simulink model "CruiseControl_System"  (R2022b)
settings: Solver=VariableStepAuto  StartTime=0.0  StopTime=100  MaxStep=0.1  RelTol=1e-3
settings Model: Creator=MAAM  LastModifiedBy=MAAM

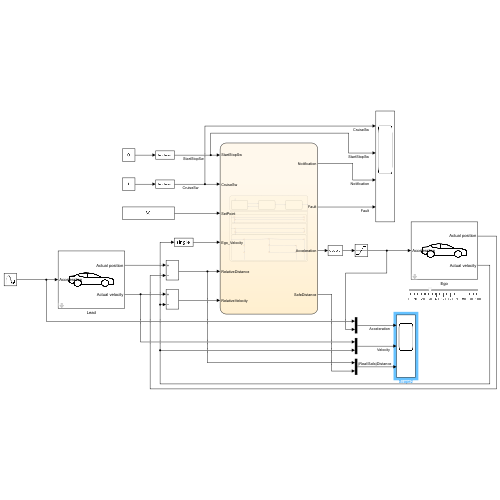
[thumbnail: Simulink's stored preview of the top-level diagram]
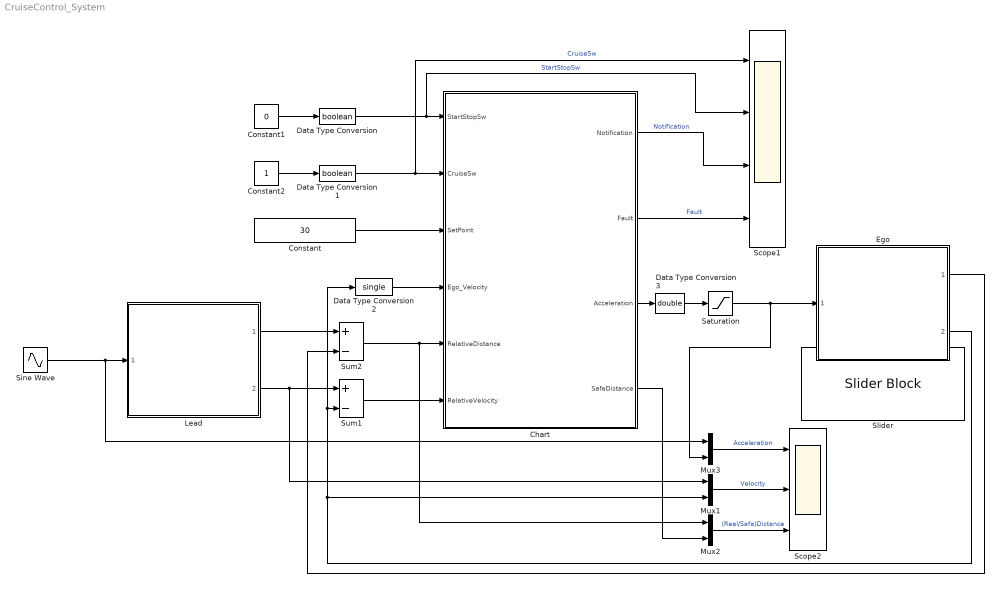
== system CruiseControl_System ==
  Chart : Stateflow chart  TreatAsAtomicUnit=on
      settings: PortSchema="{\"entries\":[{\"content\":{\"sides\":[{\"content\":{\"connectorIds\":[\"In2\",\"In1\",\"In3\",\"In4\",\"In5\",\"In6\"]},\"type\":\"ConnectorPlacement.EquallySpacedRectSide\",\"uuid\":\"a558f2c2-5ffb-4ba0-8891-a688bb62a9b9\"},{\"content\":{\"connectorIds\":[\"Out2\",\"Out1\",\"Out3\",\"Out4\"],\"side\":\"RIGHT\"},\"type\":\"ConnectorPlacement.EquallySpacedRectSide\",\"uuid\":\"56d0d55d-a484-4316-a2b8-f7c2ba28bad9\"},{\"content\":{\"connectorIds\":[],\"side\":\"TOP\"},\"type\":\"ConnectorPlacement.EquallySpacedRectSide\",\"uuid\":\"4bb91777-42b4-417b-88ce-c76e908bf247\"}]},\"type\":\"ConnectorPlacement.EquallySpacedConnector\",\"uuid\":\"a190dafd-ffc5-4ff1-968b-a32c0c19da50\"}],\"packageUris\":[\"http://schema.mathworks.com/mf0/Connector/R2020b\"],\"version\":\"1.0\"}"
  Constant : Constant  Value=30  OutDataTypeStr=single
  Constant1 : Constant  Value=0
  Constant2 : Constant
  Data Type Conversion : DataTypeConversion  OutDataTypeStr=boolean  SaturateOnIntegerOverflow=off  RndMeth=Floor
  Data Type Conversion1 : DataTypeConversion  OutDataTypeStr=boolean  SaturateOnIntegerOverflow=off  RndMeth=Floor
  Data Type Conversion2 : DataTypeConversion  OutDataTypeStr=single  SaturateOnIntegerOverflow=off  RndMeth=Floor
  Data Type Conversion3 : DataTypeConversion  OutDataTypeStr=double  SaturateOnIntegerOverflow=off  RndMeth=Floor
  Ego : Subsystem  ReferencedSubsystem=Car  InitPos=10  InitVol=20
  Lead : Subsystem  ReferencedSubsystem=Car  InitPos=50  InitVol=25
  Mux1 : Mux  Inputs=2
  Mux2 : Mux  Inputs=2
  Mux3 : Mux  Inputs=2
  Saturation : Saturate  UpperLimit=2  LowerLimit=-3
  Scope1 : Scope  NumInputPorts=4
  Scope2 : Scope  NumInputPorts=3
  Sine Wave : Sin  Amplitude=0.8  Frequency=0.2  SampleTime=0.1
  Slider : SliderBlock
  Sum1 : Sum  Inputs=+-  OutDataTypeStr=single
  Sum2 : Sum  Inputs=+-  OutDataTypeStr=single
  wires:
  Sine Wave/1 -> Mux3/1, Lead/1
  Ego/2 -> Data Type Conversion2/1, Sum1/2, Mux1/2
  Lead/2 -> Mux1/1, Sum1/1
  Lead/1 -> Sum2/1
  Ego/1 -> Sum2/2
  Mux3/1 -> Scope2/1  "Acceleration"
  Chart/2(Notification) -> Scope1/3  "Notification"
  Chart/1(Fault) -> Scope1/4  "Fault"
  Mux1/1 -> Scope2/2  "Velocity"
  Mux2/1 -> Scope2/3  "(Real/Safa)Distance"
  Data Type Conversion/1 -> Scope1/2, Chart/2(StartStopSw)  "StartStopSw"
  Data Type Conversion1/1 -> Scope1/1, Chart/1(CruiseSw)  "CruiseSw"
  Constant/1 -> Chart/3(SetPoint)
  Sum2/1 -> Mux2/1, Chart/5(RelativeDistance)
  Sum1/1 -> Chart/6(RelativeVelocity)
  Chart/4(SafeDistance) -> Mux2/2
  Data Type Conversion2/1 -> Chart/4(Ego_Velocity)
  Constant1/1 -> Data Type Conversion/1
  Constant2/1 -> Data Type Conversion1/1
  Saturation/1 -> Ego/1, Mux3/2
  Chart/3(Acceleration) -> Data Type Conversion3/1
  Data Type Conversion3/1 -> Saturation/1

== stateflow chart CruiseControl_System/Chart ==
  state Fault_Detection_Sysytem [parallel]
    settings: executionOrder=2
    state Init
      en:
      Fault = false;
      Notification = CCS_Mode.Do_Nothing;
    state Wait
      en:
      Notification = CCS_Mode.Stop;
    state Fault
      en:
      Fault = true;
      Notification = CCS_Mode.Stop;
    (default) -> Init
    Init -> Wait : FaultEvent
    Wait -> Fault [order 2] : after(FaultTime, sec)
    Fault -> Fault_Detection_Sysytem : ClearEvent
    Wait -> Init [order 1] : ClearEvent
  state Regular_System [parallel]
    settings: executionOrder=1
    state CruiseControl_Activation [parallel]
      settings: executionOrder=1
      CruiseControl_Activation -> (junction 59)
      (junction 59) -> (junction 64) [order 1] : [StartStopSw]
      (junction 59) -> (junction 62) [order 2]
      (junction 64) -> (junction 66) : {Acceleration = 0;}
      (junction 66) -> (junction 62)
      (junction 62) -> CruiseControl_Activation
    state Distance_Measurement [parallel]
      en,du:
      SafeDistance = DefaultDistance + TimeGap * Ego_Velocity;
      settings: executionOrder=2
      Distance_Measurement -> (junction 83)
      (junction 83) -> (junction 85) [order 1] : [RelativeDistance >= SafeDistance]
      (junction 83) -> (junction 89) [order 2] : {send(FaultEvent, Fault_Detection_Sysytem)}
      (junction 85) -> (junction 94) : {send(ClearEvent, Fault_Detection_Sysytem)}
      (junction 94) -> (junction 89)
      (junction 89) -> Distance_Measurement
    state CruiseControl_Operation [parallel]
      settings: executionOrder=3
      (junction 71) -> (junction 105) [order 1] : [(RelativeDistance - SafeDistance) >= DefaultDistance]
      (junction 105) -> (junction 99) [order 1] : [abs(SetPoint - Ego_Velocity) <= threshold]
      CruiseControl_Operation -> (junction 71) : [CruiseSw && ~StartStopSw]
      (junction 105) -> (junction 108) [order 2]
      (junction 71) -> (junction 138) [order 2]
      (junction 99) -> (junction 103) : {Mode = CCS_Mode.Do_Nothing;}
      (junction 108) -> (junction 110) [order 1] : [SetPoint > Ego_Velocity]
      (junction 108) -> (junction 141) [order 2] : {Mode = CCS_Mode.Decelerate;}
      (junction 138) -> (junction 120) : {Mode = CCS_Mode.Decelerate;}
      (junction 110) -> (junction 112) : {Mode = CCS_Mode.Accelerate;}
      (junction 141) -> (junction 112)
      (junction 120) -> CruiseControl_Operation : {Acceleration = ((RelativeVelocity + RelativeDistance) - SafeDistance - DefaultDistance) * 0.1;}
      (junction 112) -> CruiseControl_Operation : {Acceleration = (SetPoint - Ego_Velocity);}
      (junction 103) -> CruiseControl_Operation : {Acceleration = 0;}
  data: CruiseSw input boolean size=1; StartStopSw input boolean size=1; SetPoint input single size=1; Ego_Velocity input single size=1; RelativeDistance input single size=1; Fault output boolean size=1; FaultTime constant single =4; RelativeVelocity input single size=1; Notification output Enum: CCS_Mode size=1; TimeGap constant single =1.4; Acceleration output single size=1; SafeDistance output single size=1; DefaultDistance constant double =10; threshold constant double =0.0001; Mode local size=1
  events: FaultEvent local FUNCTION_CALL_EVENT; ClearEvent local FUNCTION_CALL_EVENT
